simulink model "dig_int_kurt"  (Simulink 6.2)
settings: Solver=ode45  StartTime=0.0  StopTime=1  RelTol=1e-3
undefined symbols (not defined in the file): bit_rev, iBOB, pfb_coeff_gen_calc
libraries: xbsIndex_r3 x1084, casper_library x95, xps_library x32
(part 4 of 8)

== system dig_int_kurt/vacc2/vacc_core2 ==
  note: This BRAM and counter is exactly what is inside the green
      | Delay BRAM block. The functionality was extracted to avoid
      | library issues.
  din : Inport  Port=1  LatchInput=off
  acc_en : Inport  Port=2  LatchInput=off
  Adder : xbsIndex_r3/AddSub  mode=Addition  precision=User Defined  arith_type=Unsigned  n_bits=48  bin_pt=23  quantization=Truncate  overflow=Wrap  latency=2  explicit_period=on  period=1  use_carryin=off  use_carryout=off  en=off  dbl_ovrd=off  show_param=on  use_core=on  pipeline=on  use_rpm=on  gen_core=off
      settings: xl_area=[0, 0, 0, 0, 0, 0, 0]
  BRAM : xbsIndex_r3/Single Port RAM  depth=1024  initVector=0  write_mode=Read Before Write  latency=2  init_zero=on  explicit_period=off  period=1  rst=off  init_reg=0  en=off  dbl_ovrd=off  show_param=off  distributed_mem=off  use_rpm=off  gen_core=off
      settings: xl_area=[0, 0, 0, 0, 0, 0, 0]
  Constant : xbsIndex_r3/Constant  const=0  equ=P=C  arith_type=Unsigned  n_bits=1  bin_pt=0  opselect=C  inp2=PCIN>>17  opr=+  inp1=P  carry=CIN  iostate=0  explicit_period=off  period=1  dbl_ovrd=off
  Constant2 : xbsIndex_r3/Constant  const=1  equ=P=C  arith_type=Boolean  n_bits=1  bin_pt=0  opselect=C  inp2=PCIN>>17  opr=+  inp1=P  carry=CIN  iostate=0  explicit_period=on  period=1  dbl_ovrd=off
  Counter : xbsIndex_r3/Counter  cnt_type=Count Limited  n_bits=10  bin_pt=0  arith_type=Unsigned  start_count=0  cnt_to=1018  cnt_by_val=1  operation=Up  explicit_period=off  period=1  load_pin=off  rst=off  en=off  dbl_ovrd=off  show_param=off  use_rpm=off  gen_core=on
      settings: xl_area=[0, 0, 0, 0, 0, 0, 0]
  Mux : xbsIndex_r3/Mux  inputs=2  precision=Full  arith_type="Signed  (2's comp)"  n_bits=8  bin_pt=2  quantization=Truncate  overflow=Wrap  latency=1  explicit_period=off  period=1  en=off  dbl_ovrd=off  show_param=on  mux_type=off  use_rpm=on  gen_core=off
      settings: xl_area=[0, 0, 0, 0, 0, 0, 0]
  dout : Outport
  wires:
  acc_en/1 -> Mux/1
  Constant/1 -> Mux/2
  BRAM/1 -> Mux/3
  din/1 -> Adder/1
  Mux/1 -> Adder/2
  Adder/1 -> dout/1, BRAM/2
  Counter/1 -> BRAM/1
  Constant2/1 -> BRAM/3

== system dig_int_kurt/fft/fft_biplex0/biplex_core ==
  pol1 : Inport  Port=1  LatchInput=off
  pol2 : Inport  Port=2  LatchInput=off
  sync : Inport  Port=3  LatchInput=off
  shift : Inport  Port=4  LatchInput=off
  fft_stage_1 : Subsystem  mask(fft_stage_n){FFTSize=10, FFTStage=1, BitWidth=18, use_bram=1, CoeffBram=0, MaxCoeffNum=16, quantization=Truncate, overflow=Wrap, add_latency=3, mult_latency=4, bram_latency=3}
      mask prompts: FFTSize "Size of FFT: (2^? pnts)"; FFTStage "Stage of FFT:"; BitWidth "Output Bitwidth:"; use_bram "Implement Delays in BRAM:"; CoeffBram "Store Coefficients in BRAM:"; MaxCoeffNum "Maximum Coefficient Depth: (2^?)"; quantization "Quantization Behavior"; overflow "Overflow Behavior"; add_latency "Add Latency"; mult_latency "Mult Latency"; bram_latency "BRAM Latency"
      mask init:
      | fft_stage_n_init(gcb,...
      |     'FFTSize', FFTSize,...
      |     'FFTStage', FFTStage,...
      |     'BitWidth', BitWidth,...
      |     'use_bram', use_bram,...
      |     'CoeffBram', CoeffBram,...
      |     'MaxCoeffNum', MaxCoeffNum,...
      |     'quantization', quantization,...
      |     'overflow', overflow,...
      |     'add_latency', add_latency,...
      |     'mult_latency', mult_latency,...
      |     'bram_latency', bram_latency);
      settings: AttributesFormatString=FFTSize=10, FFTStage=1, BitWidth=18
      mask StyleString: edit,edit,edit,edit,edit,edit,popup(Truncate|Round  (unbiased: +/- Inf)|Round  (unbiased: Even Values)),popup(Wrap|Saturate|Error),edit,edit,edit
  fft_stage_10 : Subsystem  AncestorBlock=casper_library/FFTs/fft_stage_n  mask(fft_stage_n){FFTSize=10, FFTStage=10, BitWidth=18, use_bram=0, CoeffBram=1, MaxCoeffNum=16, quantization=Truncate, overflow=Wrap, add_latency=3, mult_latency=4, bram_latency=3}
      mask prompts: FFTSize "Size of FFT: (2^? pnts)"; FFTStage "Stage of FFT:"; BitWidth "Output Bitwidth:"; use_bram "Implement Delays in BRAM:"; CoeffBram "Store Coefficients in BRAM:"; MaxCoeffNum "Maximum Coefficient Depth: (2^?)"; quantization "Quantization Behavior"; overflow "Overflow Behavior"; add_latency "Add Latency"; mult_latency "Mult Latency"; bram_latency "BRAM Latency"
      mask init: same as dig_int_kurt/fft/fft_biplex0/biplex_core/fft_stage_1
      settings: AttributesFormatString=FFTSize=10, FFTStage=10, BitWidth=18
      mask StyleString: edit,edit,edit,edit,edit,edit,popup(Truncate|Round  (unbiased: +/- Inf)|Round  (unbiased: Even Values)),popup(Wrap|Saturate|Error),edit,edit,edit
  fft_stage_2 : Subsystem  AncestorBlock=casper_library/FFTs/fft_stage_n  mask(fft_stage_n){FFTSize=10, FFTStage=2, BitWidth=18, use_bram=1, CoeffBram=0, MaxCoeffNum=16, quantization=Truncate, overflow=Wrap, add_latency=3, mult_latency=4, bram_latency=3}
      mask prompts: FFTSize "Size of FFT: (2^? pnts)"; FFTStage "Stage of FFT:"; BitWidth "Output Bitwidth:"; use_bram "Implement Delays in BRAM:"; CoeffBram "Store Coefficients in BRAM:"; MaxCoeffNum "Maximum Coefficient Depth: (2^?)"; quantization "Quantization Behavior"; overflow "Overflow Behavior"; add_latency "Add Latency"; mult_latency "Mult Latency"; bram_latency "BRAM Latency"
      mask init: same as dig_int_kurt/fft/fft_biplex0/biplex_core/fft_stage_1
      settings: AttributesFormatString=FFTSize=10, FFTStage=2, BitWidth=18
      mask StyleString: edit,edit,edit,edit,edit,edit,popup(Truncate|Round  (unbiased: +/- Inf)|Round  (unbiased: Even Values)),popup(Wrap|Saturate|Error),edit,edit,edit
  fft_stage_3 : Subsystem  AncestorBlock=casper_library/FFTs/fft_stage_n  mask(fft_stage_n){FFTSize=10, FFTStage=3, BitWidth=18, use_bram=1, CoeffBram=0, MaxCoeffNum=16, quantization=Truncate, overflow=Wrap, add_latency=3, mult_latency=4, bram_latency=3}
      mask prompts: FFTSize "Size of FFT: (2^? pnts)"; FFTStage "Stage of FFT:"; BitWidth "Output Bitwidth:"; use_bram "Implement Delays in BRAM:"; CoeffBram "Store Coefficients in BRAM:"; MaxCoeffNum "Maximum Coefficient Depth: (2^?)"; quantization "Quantization Behavior"; overflow "Overflow Behavior"; add_latency "Add Latency"; mult_latency "Mult Latency"; bram_latency "BRAM Latency"
      mask init: same as dig_int_kurt/fft/fft_biplex0/biplex_core/fft_stage_1
      settings: AttributesFormatString=FFTSize=10, FFTStage=3, BitWidth=18
      mask StyleString: edit,edit,edit,edit,edit,edit,popup(Truncate|Round  (unbiased: +/- Inf)|Round  (unbiased: Even Values)),popup(Wrap|Saturate|Error),edit,edit,edit
  fft_stage_4 : Subsystem  AncestorBlock=casper_library/FFTs/fft_stage_n  mask(fft_stage_n){FFTSize=10, FFTStage=4, BitWidth=18, use_bram=1, CoeffBram=0, MaxCoeffNum=16, quantization=Truncate, overflow=Wrap, add_latency=3, mult_latency=4, bram_latency=3}
      mask prompts: FFTSize "Size of FFT: (2^? pnts)"; FFTStage "Stage of FFT:"; BitWidth "Output Bitwidth:"; use_bram "Implement Delays in BRAM:"; CoeffBram "Store Coefficients in BRAM:"; MaxCoeffNum "Maximum Coefficient Depth: (2^?)"; quantization "Quantization Behavior"; overflow "Overflow Behavior"; add_latency "Add Latency"; mult_latency "Mult Latency"; bram_latency "BRAM Latency"
      mask init: same as dig_int_kurt/fft/fft_biplex0/biplex_core/fft_stage_1
      settings: AttributesFormatString=FFTSize=10, FFTStage=4, BitWidth=18
      mask StyleString: edit,edit,edit,edit,edit,edit,popup(Truncate|Round  (unbiased: +/- Inf)|Round  (unbiased: Even Values)),popup(Wrap|Saturate|Error),edit,edit,edit
  fft_stage_5 : Subsystem  AncestorBlock=casper_library/FFTs/fft_stage_n  mask(fft_stage_n){FFTSize=10, FFTStage=5, BitWidth=18, use_bram=0, CoeffBram=0, MaxCoeffNum=16, quantization=Truncate, overflow=Wrap, add_latency=3, mult_latency=4, bram_latency=3}
      mask prompts: FFTSize "Size of FFT: (2^? pnts)"; FFTStage "Stage of FFT:"; BitWidth "Output Bitwidth:"; use_bram "Implement Delays in BRAM:"; CoeffBram "Store Coefficients in BRAM:"; MaxCoeffNum "Maximum Coefficient Depth: (2^?)"; quantization "Quantization Behavior"; overflow "Overflow Behavior"; add_latency "Add Latency"; mult_latency "Mult Latency"; bram_latency "BRAM Latency"
      mask init: same as dig_int_kurt/fft/fft_biplex0/biplex_core/fft_stage_1
      settings: AttributesFormatString=FFTSize=10, FFTStage=5, BitWidth=18
      mask StyleString: edit,edit,edit,edit,edit,edit,popup(Truncate|Round  (unbiased: +/- Inf)|Round  (unbiased: Even Values)),popup(Wrap|Saturate|Error),edit,edit,edit
  fft_stage_6 : Subsystem  AncestorBlock=casper_library/FFTs/fft_stage_n  mask(fft_stage_n){FFTSize=10, FFTStage=6, BitWidth=18, use_bram=0, CoeffBram=0, MaxCoeffNum=16, quantization=Truncate, overflow=Wrap, add_latency=3, mult_latency=4, bram_latency=3}
      mask prompts: FFTSize "Size of FFT: (2^? pnts)"; FFTStage "Stage of FFT:"; BitWidth "Output Bitwidth:"; use_bram "Implement Delays in BRAM:"; CoeffBram "Store Coefficients in BRAM:"; MaxCoeffNum "Maximum Coefficient Depth: (2^?)"; quantization "Quantization Behavior"; overflow "Overflow Behavior"; add_latency "Add Latency"; mult_latency "Mult Latency"; bram_latency "BRAM Latency"
      mask init: same as dig_int_kurt/fft/fft_biplex0/biplex_core/fft_stage_1
      settings: AttributesFormatString=FFTSize=10, FFTStage=6, BitWidth=18
      mask StyleString: edit,edit,edit,edit,edit,edit,popup(Truncate|Round  (unbiased: +/- Inf)|Round  (unbiased: Even Values)),popup(Wrap|Saturate|Error),edit,edit,edit
  fft_stage_7 : Subsystem  AncestorBlock=casper_library/FFTs/fft_stage_n  mask(fft_stage_n){FFTSize=10, FFTStage=7, BitWidth=18, use_bram=0, CoeffBram=0, MaxCoeffNum=16, quantization=Truncate, overflow=Wrap, add_latency=3, mult_latency=4, bram_latency=3}
      mask prompts: FFTSize "Size of FFT: (2^? pnts)"; FFTStage "Stage of FFT:"; BitWidth "Output Bitwidth:"; use_bram "Implement Delays in BRAM:"; CoeffBram "Store Coefficients in BRAM:"; MaxCoeffNum "Maximum Coefficient Depth: (2^?)"; quantization "Quantization Behavior"; overflow "Overflow Behavior"; add_latency "Add Latency"; mult_latency "Mult Latency"; bram_latency "BRAM Latency"
      mask init: same as dig_int_kurt/fft/fft_biplex0/biplex_core/fft_stage_1
      settings: AttributesFormatString=FFTSize=10, FFTStage=7, BitWidth=18
      mask StyleString: edit,edit,edit,edit,edit,edit,popup(Truncate|Round  (unbiased: +/- Inf)|Round  (unbiased: Even Values)),popup(Wrap|Saturate|Error),edit,edit,edit
  fft_stage_8 : Subsystem  AncestorBlock=casper_library/FFTs/fft_stage_n  mask(fft_stage_n){FFTSize=10, FFTStage=8, BitWidth=18, use_bram=0, CoeffBram=1, MaxCoeffNum=16, quantization=Truncate, overflow=Wrap, add_latency=3, mult_latency=4, bram_latency=3}
      mask prompts: FFTSize "Size of FFT: (2^? pnts)"; FFTStage "Stage of FFT:"; BitWidth "Output Bitwidth:"; use_bram "Implement Delays in BRAM:"; CoeffBram "Store Coefficients in BRAM:"; MaxCoeffNum "Maximum Coefficient Depth: (2^?)"; quantization "Quantization Behavior"; overflow "Overflow Behavior"; add_latency "Add Latency"; mult_latency "Mult Latency"; bram_latency "BRAM Latency"
      mask init: same as dig_int_kurt/fft/fft_biplex0/biplex_core/fft_stage_1
      settings: AttributesFormatString=FFTSize=10, FFTStage=8, BitWidth=18
      mask StyleString: edit,edit,edit,edit,edit,edit,popup(Truncate|Round  (unbiased: +/- Inf)|Round  (unbiased: Even Values)),popup(Wrap|Saturate|Error),edit,edit,edit
  fft_stage_9 : Subsystem  AncestorBlock=casper_library/FFTs/fft_stage_n  mask(fft_stage_n){FFTSize=10, FFTStage=9, BitWidth=18, use_bram=0, CoeffBram=1, MaxCoeffNum=16, quantization=Truncate, overflow=Wrap, add_latency=3, mult_latency=4, bram_latency=3}
      mask prompts: FFTSize "Size of FFT: (2^? pnts)"; FFTStage "Stage of FFT:"; BitWidth "Output Bitwidth:"; use_bram "Implement Delays in BRAM:"; CoeffBram "Store Coefficients in BRAM:"; MaxCoeffNum "Maximum Coefficient Depth: (2^?)"; quantization "Quantization Behavior"; overflow "Overflow Behavior"; add_latency "Add Latency"; mult_latency "Mult Latency"; bram_latency "BRAM Latency"
      mask init: same as dig_int_kurt/fft/fft_biplex0/biplex_core/fft_stage_1
      settings: AttributesFormatString=FFTSize=10, FFTStage=9, BitWidth=18
      mask StyleString: edit,edit,edit,edit,edit,edit,popup(Truncate|Round  (unbiased: +/- Inf)|Round  (unbiased: Even Values)),popup(Wrap|Saturate|Error),edit,edit,edit
  out1 : Outport
  out2 : Outport  Port=2
  of : Outport  Port=3
  sync_out : Outport  Port=4
  wires:
  fft_stage_1/1(out1) -> fft_stage_2/1(in1)
  fft_stage_1/2(out2) -> fft_stage_2/2(in2)
  fft_stage_1/3(of) -> fft_stage_2/3(of_in)
  fft_stage_1/4(sync_out) -> fft_stage_2/4(sync)
  shift/1 -> fft_stage_2/5(shift), fft_stage_3/5(shift), fft_stage_4/5(shift), fft_stage_5/5(shift), fft_stage_6/5(shift), fft_stage_7/5(shift), fft_stage_8/5(shift), fft_stage_9/5(shift), fft_stage_10/5(shift), fft_stage_1/4(shift)
  fft_stage_2/1(out1) -> fft_stage_3/1(in1)
  fft_stage_2/2(out2) -> fft_stage_3/2(in2)
  fft_stage_2/3(of) -> fft_stage_3/3(of_in)
  fft_stage_2/4(sync_out) -> fft_stage_3/4(sync)
  fft_stage_3/1(out1) -> fft_stage_4/1(in1)
  fft_stage_3/2(out2) -> fft_stage_4/2(in2)
  fft_stage_3/3(of) -> fft_stage_4/3(of_in)
  fft_stage_3/4(sync_out) -> fft_stage_4/4(sync)
  fft_stage_4/1(out1) -> fft_stage_5/1(in1)
  fft_stage_4/2(out2) -> fft_stage_5/2(in2)
  fft_stage_4/3(of) -> fft_stage_5/3(of_in)
  fft_stage_4/4(sync_out) -> fft_stage_5/4(sync)
  fft_stage_5/1(out1) -> fft_stage_6/1(in1)
  fft_stage_5/2(out2) -> fft_stage_6/2(in2)
  fft_stage_5/3(of) -> fft_stage_6/3(of_in)
  fft_stage_5/4(sync_out) -> fft_stage_6/4(sync)
  fft_stage_6/1(out1) -> fft_stage_7/1(in1)
  fft_stage_6/2(out2) -> fft_stage_7/2(in2)
  fft_stage_6/3(of) -> fft_stage_7/3(of_in)
  fft_stage_6/4(sync_out) -> fft_stage_7/4(sync)
  fft_stage_7/1(out1) -> fft_stage_8/1(in1)
  fft_stage_7/2(out2) -> fft_stage_8/2(in2)
  fft_stage_7/3(of) -> fft_stage_8/3(of_in)
  fft_stage_7/4(sync_out) -> fft_stage_8/4(sync)
  fft_stage_8/1(out1) -> fft_stage_9/1(in1)
  fft_stage_8/2(out2) -> fft_stage_9/2(in2)
  fft_stage_8/3(of) -> fft_stage_9/3(of_in)
  fft_stage_8/4(sync_out) -> fft_stage_9/4(sync)
  fft_stage_9/1(out1) -> fft_stage_10/1(in1)
  fft_stage_9/2(out2) -> fft_stage_10/2(in2)
  fft_stage_9/3(of) -> fft_stage_10/3(of_in)
  fft_stage_9/4(sync_out) -> fft_stage_10/4(sync)
  pol1/1 -> fft_stage_1/1(in1)
  pol2/1 -> fft_stage_1/2(in2)
  sync/1 -> fft_stage_1/3(sync)
  fft_stage_10/1(out1) -> out1/1
  fft_stage_10/2(out2) -> out2/1
  fft_stage_10/3(of) -> of/1
  fft_stage_10/4(sync_out) -> sync_out/1

== system dig_int_kurt/fft/fft_biplex0/biplex_cplx_unscrambler ==
  even : Inport  Port=1  LatchInput=off
  odd : Inport  Port=2  LatchInput=off
  sync : Inport  Port=3  LatchInput=off
  Constant : xbsIndex_r3/Constant  const=1  equ=P=C  arith_type=Boolean  n_bits=1  bin_pt=0  opselect=C  inp2=PCIN>>17  opr=+  inp1=P  carry=CIN  iostate=0  explicit_period=on  period=1  dbl_ovrd=off
  Constant1 : xbsIndex_r3/Constant  const=2^(FFTSize-1)  equ=P=C  arith_type=Unsigned  n_bits=FFTSize  bin_pt=0  opselect=C  inp2=PCIN>>17  opr=+  inp1=P  carry=CIN  iostate=0  explicit_period=on  period=1  dbl_ovrd=off
  Constant2 : xbsIndex_r3/Constant  const=2^(FFTSize-1)  equ=P=C  arith_type=Unsigned  n_bits=FFTSize  bin_pt=0  opselect=C  inp2=PCIN>>17  opr=+  inp1=P  carry=CIN  iostate=0  explicit_period=on  period=1  dbl_ovrd=off
  Convert : xbsIndex_r3/Convert  arith_type=Unsigned  n_bits=1  bin_pt=0  quantization=Truncate  overflow=Wrap  latency=0  explicit_period=off  period=1  dbl_ovrd=off  show_param=off  inserted_by_tool=off  pipeline=off
      settings: xl_area=[0, 0, 0, 0, 0, 0, 0]
  Convert1 : xbsIndex_r3/Convert  arith_type=Unsigned  n_bits=1  bin_pt=0  quantization=Truncate  overflow=Wrap  latency=0  explicit_period=off  period=1  dbl_ovrd=off  show_param=off  inserted_by_tool=off  pipeline=off
      settings: xl_area=[0, 0, 0, 0, 0, 0, 0]
  Counter : xbsIndex_r3/Counter  cnt_type=Free Running  n_bits=FFTSize  bin_pt=0  arith_type=Unsigned  start_count=0  cnt_to=Inf  cnt_by_val=1  operation=Up  explicit_period=off  period=1  load_pin=off  rst=on  en=off  dbl_ovrd=off  show_param=off  use_rpm=on  gen_core=off
      settings: xl_area=[0, 0, 0, 0, 0, 0, 0]
  Counter1 : xbsIndex_r3/Counter  cnt_type=Free Running  n_bits=FFTSize  bin_pt=0  arith_type=Unsigned  start_count=0  cnt_to=Inf  cnt_by_val=1  operation=Up  explicit_period=off  period=1  load_pin=off  rst=on  en=off  dbl_ovrd=off  show_param=off  use_rpm=on  gen_core=off
      settings: xl_area=[0, 0, 0, 0, 0, 0, 0]
  Relational : xbsIndex_r3/Relational  mode=a<=b  latency=0  explicit_period=off  period=1  en=off  dbl_ovrd=off  show_param=off
      settings: xl_area=[0, 0, 0, 0, 0, 0, 0]
  Relational1 : xbsIndex_r3/Relational  mode=a<=b  latency=0  explicit_period=off  period=1  en=off  dbl_ovrd=off  show_param=off
      settings: xl_area=[0, 0, 0, 0, 0, 0, 0]
  barrel_switcher : Subsystem  AncestorBlock=casper_library/Reorder/barrel_switcher  mask(barrel_switcher){n_inputs=1}
      mask prompts: n_inputs "Number of Inputs: (2^?)"
      mask init:
      | barrel_switcher_init(gcb,...
      |     'n_inputs', n_inputs);
      settings: AttributesFormatString=n_inputs=1
  barrel_switcher1 : Subsystem  AncestorBlock=casper_library/Reorder/barrel_switcher  mask(barrel_switcher){n_inputs=1}
      mask prompts: n_inputs "Number of Inputs: (2^?)"
      mask init:
      | barrel_switcher_init(gcb,...
      |     'n_inputs', n_inputs);
      settings: AttributesFormatString=n_inputs=1
  reorder : Subsystem  AncestorBlock=casper_library/Reorder/reorder  mask(reorder){map=[0 256 128 384 64 320 192 448 32 288 160 416 96 352 224 480 16 272 144 400 80 336 208 464 48 304 176 432 112 368 240 496 8 264 136 392 72 328 200 456 40 296 168 424 104 360 232 488 24 280 152 408 88 344 216 472 56 312 184 440 120 376 248 504 4 260 132 388 68 324 196 452 36 292 164 420 100 356 228 484 20 276 148 404 84 340 212 468 52 308 180 436 116 372 244 500 12 268 140 396 76 332 204 460 44 300 172 428 108 364 236 492 28 284 156 412 92 348 220 476 60 316 188 444 124 380 252 508 2 258 130 386 66 322 194 450 34 290 162 418 98 354 226 482 18 274 146 402 82 338 210 466 50 306 178 434 114 370 242 498 10 266 138 394 74 330 202 458 42 298 170 426 106 362 234 490 26 282 154 410 90 346 218 474 58 314 186 442 122 378 250 506 6 262 134 390 70 326 198 454 38 294 166 422 102 358 230 486 22 278 150 406 86 342 214 470 54 310 182 438 118 374 246 502 14 270 142 398 78 334 206 462 46 302 174 430 110 366 238 494 30 286 158 414 94 350 222 478 62 318 190 446 126 382 254 510 1 257 129 385 65 321 193 449 33 289 161 417 97 353 225 481 17 273 145 401 81 337 209 465 49 305 177 433 113 369 241 497 9 265 137 393 73 329 201 457 41 297 169 425 105 361 233 489 25 281 153 409 89 345 217 473 57 313 185 441 121 377 249 505 5 261 133 389 69 325 197 453 37 293 165 421 101 357 229 485 21 277 149 405 85 341 213 469 53 309 181 437 117 373 245 501 13 269 141 397 77 333 205 461 45 301 173 429 109 365 237 493 29 285 157 413 93 349 221 477 61 317 189 445 125 381 253 509 3 259 131 387 67 323 195 451 35 291 163 419 99 355 227 483 19 275 147 403 83 339 211 467 51 307 179 435 115 371 243 499 11 267 139 395 75 331 203 459 43 299 171 427 107 363 235 491 27 283 155 411 91 347 219 475 59 315 187 443 123 379 251 507 7 263 135 391 71 327 199 455 39 295 167 423 103 359 231 487 23 279 151 407 87 343 215 471 55 311 183 439 119 375 247 503 15 271 143 399 79 335 207 463 47 303 175 431 111 367 239 495 31 287 159 415 95 351 223 479 63 319 191 447 127 383 255 511 512 768 640 896 576 832 704 960 544 800 672 928 608 864 736 992 528 784 656 912 592 848 720 976 560 816 688 944 624 880 752 1008 520 776 648 904 584 840 712 968 552 808 680 936 616 872 744 1000 536 792 664 920 600 856 728 984 568 824 696 952 632 888 760 1016 516 772 644 900 580 836 708 964 548 804 676 932 612 868 740 996 532 788 660 916 596 852 724 980 564 820 692 948 628 884 756 1012 524 780 652 908 588 844 716 972 556 812 684 940 620 876 748 1004 540 796 668 924 604 860 732 988 572 828 700 956 636 892 764 1020 514 770 642 898 578 834 706 962 546 802 674 930 610 866 738 994 530 786 658 914 594 850 722 978 562 818 690 946 626 882 754 1010 522 778 650 906 586 842 714 970 554 810 682 938 618 874 746 1002 538 794 666 922 602 858 730 986 570 826 698 954 634 890 762 1018 518 774 646 902 582 838 710 966 550 806 678 934 614 870 742 998 534 790 662 918 598 854 726 982 566 822 694 950 630 886 758 1014 526 782 654 910 590 846 718 974 558 814 686 942 622 878 750 1006 542 798 670 926 606 862 734 990 574 830 702 958 638 894 766 1022 513 769 641 897 577 833 705 961 545 801 673 929 609 865 737 993 529 785 657 913 593 849 721 977 561 817 689 945 625 881 753 1009 521 777 649 905 585 841 713 969 553 809 681 937 617 873 745 1001 537 793 665 921 601 857 729 985 569 825 697 953 633 889 761 1017 517 773 645 901 581 837 709 965 549 805 677 933 613 869 741 997 533 789 661 917 597 853 725 981 565 821 693 949 629 885 757 1013 525 781 653 909 589 845 717 973 557 813 685 941 621 877 749 1005 541 797 669 925 605 861 733 989 573 829 701 957 637 893 765 1021 515 771 643 899 579 835 707 963 547 803 675 931 611 867 739 995 531 787 659 915 595 851 723 979 563 819 691 947 627 883 755 1011 523 779 651 907 587 843 715 971 555 811 683 939 619 875 747 1003 539 795 667 923 603 859 731 987 571 827 699 955 635 891 763 1019 519 775 647 903 583 839 711 967 551 807 679 935 615 871 743 999 535 791 663 919 599 855 727 983 567 823 695 951 631 887 759 1015 527 783 655 911 591 847 719 975 559 815 687 943 623 879 751 1007 543 799 671 927 607 863 735 991 575 831 703 959 639 895 767 1023], n_inputs=1, bram_latency=3, map_latency=0, double_buffer=0}
      mask prompts: map "Output Order:"; n_inputs "Number of inputs"; bram_latency "BRAM Latency"; map_latency "Map Latency"; double_buffer "Double Buffer"
      mask init:
      | reorder_init(gcb, ...
      |     'map', map, ...
      |     'n_inputs', n_inputs, ...
      |     'bram_latency', bram_latency, ...
      |     'map_latency', map_latency, ...
      |     'double_buffer', double_buffer);
      settings: AttributesFormatString=order=2
  reorder1 : Subsystem  AncestorBlock=casper_library/Reorder/reorder  mask(reorder){map=[512 768 640 896 576 832 704 960 544 800 672 928 608 864 736 992 528 784 656 912 592 848 720 976 560 816 688 944 624 880 752 1008 520 776 648 904 584 840 712 968 552 808 680 936 616 872 744 1000 536 792 664 920 600 856 728 984 568 824 696 952 632 888 760 1016 516 772 644 900 580 836 708 964 548 804 676 932 612 868 740 996 532 788 660 916 596 852 724 980 564 820 692 948 628 884 756 1012 524 780 652 908 588 844 716 972 556 812 684 940 620 876 748 1004 540 796 668 924 604 860 732 988 572 828 700 956 636 892 764 1020 514 770 642 898 578 834 706 962 546 802 674 930 610 866 738 994 530 786 658 914 594 850 722 978 562 818 690 946 626 882 754 1010 522 778 650 906 586 842 714 970 554 810 682 938 618 874 746 1002 538 794 666 922 602 858 730 986 570 826 698 954 634 890 762 1018 518 774 646 902 582 838 710 966 550 806 678 934 614 870 742 998 534 790 662 918 598 854 726 982 566 822 694 950 630 886 758 1014 526 782 654 910 590 846 718 974 558 814 686 942 622 878 750 1006 542 798 670 926 606 862 734 990 574 830 702 958 638 894 766 1022 513 769 641 897 577 833 705 961 545 801 673 929 609 865 737 993 529 785 657 913 593 849 721 977 561 817 689 945 625 881 753 1009 521 777 649 905 585 841 713 969 553 809 681 937 617 873 745 1001 537 793 665 921 601 857 729 985 569 825 697 953 633 889 761 1017 517 773 645 901 581 837 709 965 549 805 677 933 613 869 741 997 533 789 661 917 597 853 725 981 565 821 693 949 629 885 757 1013 525 781 653 909 589 845 717 973 557 813 685 941 621 877 749 1005 541 797 669 925 605 861 733 989 573 829 701 957 637 893 765 1021 515 771 643 899 579 835 707 963 547 803 675 931 611 867 739 995 531 787 659 915 595 851 723 979 563 819 691 947 627 883 755 1011 523 779 651 907 587 843 715 971 555 811 683 939 619 875 747 1003 539 795 667 923 603 859 731 987 571 827 699 955 635 891 763 1019 519 775 647 903 583 839 711 967 551 807 679 935 615 871 743 999 535 791 663 919 599 855 727 983 567 823 695 951 631 887 759 1015 527 783 655 911 591 847 719 975 559 815 687 943 623 879 751 1007 543 799 671 927 607 863 735 991 575 831 703 959 639 895 767 1023 0 256 128 384 64 320 192 448 32 288 160 416 96 352 224 480 16 272 144 400 80 336 208 464 48 304 176 432 112 368 240 496 8 264 136 392 72 328 200 456 40 296 168 424 104 360 232 488 24 280 152 408 88 344 216 472 56 312 184 440 120 376 248 504 4 260 132 388 68 324 196 452 36 292 164 420 100 356 228 484 20 276 148 404 84 340 212 468 52 308 180 436 116 372 244 500 12 268 140 396 76 332 204 460 44 300 172 428 108 364 236 492 28 284 156 412 92 348 220 476 60 316 188 444 124 380 252 508 2 258 130 386 66 322 194 450 34 290 162 418 98 354 226 482 18 274 146 402 82 338 210 466 50 306 178 434 114 370 242 498 10 266 138 394 74 330 202 458 42 298 170 426 106 362 234 490 26 282 154 410 90 346 218 474 58 314 186 442 122 378 250 506 6 262 134 390 70 326 198 454 38 294 166 422 102 358 230 486 22 278 150 406 86 342 214 470 54 310 182 438 118 374 246 502 14 270 142 398 78 334 206 462 46 302 174 430 110 366 238 494 30 286 158 414 94 350 222 478 62 318 190 446 126 382 254 510 1 257 129 385 65 321 193 449 33 289 161 417 97 353 225 481 17 273 145 401 81 337 209 465 49 305 177 433 113 369 241 497 9 265 137 393 73 329 201 457 41 297 169 425 105 361 233 489 25 281 153 409 89 345 217 473 57 313 185 441 121 377 249 505 5 261 133 389 69 325 197 453 37 293 165 421 101 357 229 485 21 277 149 405 85 341 213 469 53 309 181 437 117 373 245 501 13 269 141 397 77 333 205 461 45 301 173 429 109 365 237 493 29 285 157 413 93 349 221 477 61 317 189 445 125 381 253 509 3 259 131 387 67 323 195 451 35 291 163 419 99 355 227 483 19 275 147 403 83 339 211 467 51 307 179 435 115 371 243 499 11 267 139 395 75 331 203 459 43 299 171 427 107 363 235 491 27 283 155 411 91 347 219 475 59 315 187 443 123 379 251 507 7 263 135 391 71 327 199 455 39 295 167 423 103 359 231 487 23 279 151 407 87 343 215 471 55 311 183 439 119 375 247 503 15 271 143 399 79 335 207 463 47 303 175 431 111 367 239 495 31 287 159 415 95 351 223 479 63 319 191 447 127 383 255 511], n_inputs=1, bram_latency=3, map_latency=0, double_buffer=0}
      mask prompts: map "Output Order:"; n_inputs "Number of inputs"; bram_latency "BRAM Latency"; map_latency "Map Latency"; double_buffer "Double Buffer"
      mask init:
      | reorder_init(gcb, ...
      |     'map', map, ...
      |     'n_inputs', n_inputs, ...
      |     'bram_latency', bram_latency, ...
      |     'map_latency', map_latency, ...
      |     'double_buffer', double_buffer);
      settings: AttributesFormatString=order=2
  pol1 : Outport
  pol2 : Outport  Port=2
  sync_out : Outport  Port=3
  wires:
  Convert/1 -> barrel_switcher/1(sel)
  Convert1/1 -> barrel_switcher1/1(sel)
  Relational1/1 -> Convert1/1
  Relational/1 -> Convert/1
  Constant2/1 -> Relational1/1
  Counter1/1 -> Relational1/2
  Counter/1 -> Relational/2
  Constant1/1 -> Relational/1
  Constant/1 -> reorder1/2(en), reorder/2(en)
  sync/1 -> Counter/1, barrel_switcher/2(sync_in)
  barrel_switcher1/3(Out2) -> pol2/1
  barrel_switcher1/2(Out1) -> pol1/1
  barrel_switcher1/1(sync_out) -> sync_out/1
  odd/1 -> barrel_switcher/4(In2)
  even/1 -> barrel_switcher/3(In1)
  reorder1/3(dout0) -> barrel_switcher1/4(In2)
  reorder/3(dout0) -> barrel_switcher1/3(In1)
  reorder/1(sync_out) -> Counter1/1, barrel_switcher1/2(sync_in)
  barrel_switcher/3(Out2) -> reorder1/3(din0)
  barrel_switcher/2(Out1) -> reorder/3(din0)
  barrel_switcher/1(sync_out) -> reorder1/1(sync), reorder/1(sync)

== system dig_int_kurt/pfb_fir/pol1_in1_first_tap/delay ==
  In1 : Inport  Port=1  LatchInput=off
  delay_bram : casper_library/Delays/delay_bram  DelayLen=2^(PFBSize-n_inputs)  bram_latency=bram_latency
  Out1 : Outport
  wires:
  In1/1 -> delay_bram/1
  delay_bram/1 -> Out1/1

== system dig_int_kurt/pfb_fir/pol1_in1_first_tap/pfb_coeff_gen ==
  din : Inport  Port=1  LatchInput=off
  sync : Inport  Port=2  LatchInput=off
  Concat : xbsIndex_r3/Concat  num_inputs=4  explicit_period=off  period=1  dbl_ovrd=off
  Counter : xbsIndex_r3/Counter  cnt_type=Free Running  n_bits=10  bin_pt=0  arith_type=Unsigned  start_count=0  cnt_to=Inf  cnt_by_val=1  operation=Up  explicit_period=on  period=1  load_pin=off  rst=on  en=off  dbl_ovrd=off  show_param=off  use_rpm=on  gen_core=off
      settings: xl_area=[0, 0, 0, 0, 0, 0, 0]
  Delay : xbsIndex_r3/Delay  latency=bram_latency+1  reg_retiming=off  explicit_period=off  period=1  en=off  accept_only_valid=off  init_zero=on  dbl_ovrd=off  show_param=off
      settings: xl_area=[0, 0, 0, 0, 0, 0, 0]
  Delay1 : xbsIndex_r3/Delay  latency=4  reg_retiming=off  explicit_period=off  period=1  en=off  accept_only_valid=off  init_zero=on  dbl_ovrd=off  show_param=off
      settings: xl_area=[0, 0, 0, 0, 0, 0, 0]
  ROM1 : xbsIndex_r3/ROM  depth=1024  initVector=pfb_coeff_gen_calc(10, 4,'hamming',0, 0,1,1)  arith_type="Signed  (2's comp)"  n_bits=8  bin_pt=7  latency=3  init_zero=on  explicit_period=off  period=1  rst=off  init_reg=0  en=off  dbl_ovrd=off  show_param=on  distributed_mem=on  use_rpm=on  gen_core=off
      settings: xl_area=[0, 0, 0, 0, 0, 0, 0]
  ROM2 : xbsIndex_r3/ROM  depth=1024  initVector=pfb_coeff_gen_calc(10, 4,'hamming',0, 0,1,2)  arith_type="Signed  (2's comp)"  n_bits=8  bin_pt=7  latency=3  init_zero=on  explicit_period=off  period=1  rst=off  init_reg=0  en=off  dbl_ovrd=off  show_param=on  distributed_mem=on  use_rpm=on  gen_core=off
      settings: xl_area=[0, 0, 0, 0, 0, 0, 0]
  ROM3 : xbsIndex_r3/ROM  depth=1024  initVector=pfb_coeff_gen_calc(10, 4,'hamming',0, 0,1,3)  arith_type="Signed  (2's comp)"  n_bits=8  bin_pt=7  latency=3  init_zero=on  explicit_period=off  period=1  rst=off  init_reg=0  en=off  dbl_ovrd=off  show_param=off  distributed_mem=on  use_rpm=on  gen_core=off
      settings: xl_area=[0, 0, 0, 0, 0, 0, 0]
  ROM4 : xbsIndex_r3/ROM  depth=1024  initVector=pfb_coeff_gen_calc(10, 4,'hamming',0, 0,1,4)  arith_type="Signed  (2's comp)"  n_bits=8  bin_pt=7  latency=3  init_zero=on  explicit_period=off  period=1  rst=off  init_reg=0  en=off  dbl_ovrd=off  show_param=off  distributed_mem=on  use_rpm=on  gen_core=off
      settings: xl_area=[0, 0, 0, 0, 0, 0, 0]
  Register : xbsIndex_r3/Register  init=0  reg_only_valid=off  explicit_period=off  period=1  rst=off  en=off  out_en=off  dbl_ovrd=off  show_param=off
      settings: xl_area=[0, 0, 0, 0, 0, 0, 0]
  Reinterpret{1..4} (4 alike) : xbsIndex_r3/Reinterpret  force_arith_type=on  arith_type=Unsigned  force_bin_pt=on  bin_pt=0  force_valid=on
  dout : Outport
  sync_out : Outport  Port=2
  coeff : Outport  Port=3
  wires:
  din/1 -> Delay1/1
  Delay1/1 -> dout/1
  sync/1 -> Counter/1, Delay/1
  Delay/1 -> sync_out/1
  Concat/1 -> Register/1
  Register/1 -> coeff/1
  Counter/1 -> ROM1/1, ROM2/1, ROM3/1, ROM4/1
  ROM1/1 -> Reinterpret1/1
  Reinterpret1/1 -> Concat/1
  ROM2/1 -> Reinterpret2/1
  Reinterpret2/1 -> Concat/2
  ROM3/1 -> Reinterpret3/1
  Reinterpret3/1 -> Concat/3
  ROM4/1 -> Reinterpret4/1
  Reinterpret4/1 -> Concat/4

== system dig_int_kurt/pfb_fir/pol1_in1_first_tap/ri_to_c ==
  re : Inport  Port=1  LatchInput=off
  im : Inport  Port=2  LatchInput=off
  Concat : xbsIndex_r3/Concat  num_inputs=2  explicit_period=off  period=1  dbl_ovrd=off
  Reinterpret : xbsIndex_r3/Reinterpret  force_arith_type=on  arith_type=Unsigned  force_bin_pt=on  bin_pt=0  force_valid=on
  Reinterpret1 : xbsIndex_r3/Reinterpret  force_arith_type=on  arith_type=Unsigned  force_bin_pt=on  bin_pt=0  force_valid=on
  c : Outport
  wires:
  Reinterpret/1 -> Concat/1
  Reinterpret1/1 -> Concat/2
  re/1 -> Reinterpret/1
  Concat/1 -> c/1
  im/1 -> Reinterpret1/1

== system dig_int_kurt/pfb_fir/pol1_in1_last_tap/pfb_add_tree ==
  din : Inport  Port=1  LatchInput=off
  sync : Inport  Port=2  LatchInput=off
  Reint0_1 : xbsIndex_r3/Reinterpret  force_arith_type=on  arith_type="Signed  (2's comp)"  force_bin_pt=on  bin_pt=14  force_valid=on
  Reint0_2 : xbsIndex_r3/Reinterpret  force_arith_type=on  arith_type="Signed  (2's comp)"  force_bin_pt=on  bin_pt=14  force_valid=on
  Reint1_1 : xbsIndex_r3/Reinterpret  force_arith_type=on  arith_type="Signed  (2's comp)"  force_bin_pt=on  bin_pt=14  force_valid=on
  Reint1_2 : xbsIndex_r3/Reinterpret  force_arith_type=on  arith_type="Signed  (2's comp)"  force_bin_pt=on  bin_pt=14  force_valid=on
  Reint2_1 : xbsIndex_r3/Reinterpret  force_arith_type=on  arith_type="Signed  (2's comp)"  force_bin_pt=on  bin_pt=14  force_valid=on
  Reint2_2 : xbsIndex_r3/Reinterpret  force_arith_type=on  arith_type="Signed  (2's comp)"  force_bin_pt=on  bin_pt=14  force_valid=on
  Reint3_1 : xbsIndex_r3/Reinterpret  force_arith_type=on  arith_type="Signed  (2's comp)"  force_bin_pt=on  bin_pt=14  force_valid=on
  Reint3_2 : xbsIndex_r3/Reinterpret  force_arith_type=on  arith_type="Signed  (2's comp)"  force_bin_pt=on  bin_pt=14  force_valid=on
  Slice0_1 : xbsIndex_r3/Slice  mode=Upper Bit Location + Width  nbits=16  bit1=0  base1=MSB of Input  bit0=0  base0=MSB of Input  boolean_output=off  explicit_period=off  period=1  dbl_ovrd=off
  Slice0_2 : xbsIndex_r3/Slice  mode=Upper Bit Location + Width  nbits=16  bit1=-16  base1=MSB of Input  bit0=0  base0=MSB of Input  boolean_output=off  explicit_period=off  period=1  dbl_ovrd=off
  Slice1_1 : xbsIndex_r3/Slice  mode=Upper Bit Location + Width  nbits=16  bit1=-32  base1=MSB of Input  bit0=0  base0=MSB of Input  boolean_output=off  explicit_period=off  period=1  dbl_ovrd=off
  Slice1_2 : xbsIndex_r3/Slice  mode=Upper Bit Location + Width  nbits=16  bit1=-48  base1=MSB of Input  bit0=0  base0=MSB of Input  boolean_output=off  explicit_period=off  period=1  dbl_ovrd=off
  Slice2_1 : xbsIndex_r3/Slice  mode=Upper Bit Location + Width  nbits=16  bit1=-64  base1=MSB of Input  bit0=0  base0=MSB of Input  boolean_output=off  explicit_period=off  period=1  dbl_ovrd=off
  Slice2_2 : xbsIndex_r3/Slice  mode=Upper Bit Location + Width  nbits=16  bit1=-80  base1=MSB of Input  bit0=0  base0=MSB of Input  boolean_output=off  explicit_period=off  period=1  dbl_ovrd=off
  Slice3_1 : xbsIndex_r3/Slice  mode=Upper Bit Location + Width  nbits=16  bit1=-96  base1=MSB of Input  bit0=0  base0=MSB of Input  boolean_output=off  explicit_period=off  period=1  dbl_ovrd=off
  Slice3_2 : xbsIndex_r3/Slice  mode=Upper Bit Location + Width  nbits=16  bit1=-112  base1=MSB of Input  bit0=0  base0=MSB of Input  boolean_output=off  explicit_period=off  period=1  dbl_ovrd=off
  adder_tree1 : Subsystem  AncestorBlock=casper_library/Misc/adder_tree  mask(adder_tree){n_inputs=4, latency=2}
      mask prompts: n_inputs "Number of Inputs"; latency "Add Latency"
      mask help: Sums all inputs using a tree of adds and delays.
      mask init:
      | adder_tree_init(gcb, ...
      |     'n_inputs', n_inputs, ...
      |     'latency', latency);
      settings: AttributesFormatString=latency 4
      mask Help: eval('xlWeb([getenv(''MLIB_ROOT''), ''\doc\html\sp_adder_tree\sp_adder_tree.html''])')
  adder_tree2 : Subsystem  AncestorBlock=casper_library/Misc/adder_tree  mask(adder_tree){n_inputs=4, latency=2}
      mask prompts: n_inputs "Number of Inputs"; latency "Add Latency"
      mask help: Sums all inputs using a tree of adds and delays.
      mask init:
      | adder_tree_init(gcb, ...
      |     'n_inputs', n_inputs, ...
      |     'latency', latency);
      settings: AttributesFormatString=latency 4
      mask Help: eval('xlWeb([getenv(''MLIB_ROOT''), ''\doc\html\sp_adder_tree\sp_adder_tree.html''])')
  convert1 : xbsIndex_r3/Convert  arith_type="Signed  (2's comp)"  n_bits=18  bin_pt=17  quantization=Truncate  overflow=Saturate  latency=2  explicit_period=off  period=1  dbl_ovrd=off  show_param=off  inserted_by_tool=off  pipeline=off
      settings: xl_area=[0, 0, 0, 0, 0, 0, 0]
  convert2 : xbsIndex_r3/Convert  arith_type="Signed  (2's comp)"  n_bits=18  bin_pt=17  quantization=Truncate  overflow=Saturate  latency=2  explicit_period=off  period=1  dbl_ovrd=off  show_param=off  inserted_by_tool=off  pipeline=off
      settings: xl_area=[0, 0, 0, 0, 0, 0, 0]
  delay1 : xbsIndex_r3/Delay  latency=2  reg_retiming=off  explicit_period=off  period=1  en=off  accept_only_valid=off  init_zero=on  dbl_ovrd=off  show_param=off
      settings: xl_area=[0, 0, 0, 0, 0, 0, 0]
  ri_to_c : casper_library/Misc/ri_to_c
  scale1 : xbsIndex_r3/Scale  scale_factor=-3  explicit_period=off  period=1  dbl_ovrd=off
  scale2 : xbsIndex_r3/Scale  scale_factor=-3  explicit_period=off  period=1  dbl_ovrd=off
  dout : Outport
  sync_out : Outport  Port=2
  wires:
  adder_tree1/2(dout) -> scale1/1
  scale1/1 -> convert1/1
  adder_tree2/2(dout) -> scale2/1
  scale2/1 -> convert2/1
  convert1/1 -> ri_to_c/1
  convert2/1 -> ri_to_c/2
  ri_to_c/1 -> dout/1
  sync/1 -> adder_tree1/1(sync), adder_tree2/1(sync)
  adder_tree1/1(sync_out) -> delay1/1
  delay1/1 -> sync_out/1
  din/1 -> Slice0_1/1, Slice0_2/1, Slice1_1/1, Slice1_2/1, Slice2_1/1, Slice2_2/1, Slice3_1/1, Slice3_2/1
  Slice0_1/1 -> Reint0_1/1
  Reint0_1/1 -> adder_tree1/2(din1)
  Slice0_2/1 -> Reint0_2/1
  Reint0_2/1 -> adder_tree2/2(din1)
  Slice1_1/1 -> Reint1_1/1
  Reint1_1/1 -> adder_tree1/3(din2)
  Slice1_2/1 -> Reint1_2/1
  Reint1_2/1 -> adder_tree2/3(din2)
  Slice2_1/1 -> Reint2_1/1
  Reint2_1/1 -> adder_tree1/4(din3)
  Slice2_2/1 -> Reint2_2/1
  Reint2_2/1 -> adder_tree2/4(din3)
  Slice3_1/1 -> Reint3_1/1
  Reint3_1/1 -> adder_tree1/5(din4)
  Slice3_2/1 -> Reint3_2/1
  Reint3_2/1 -> adder_tree2/5(din4)

== system dig_int_kurt/pfb_fir/pol1_in1_last_tap/ri_to_c ==
  re : Inport  Port=1  LatchInput=off
  im : Inport  Port=2  LatchInput=off
  Concat : xbsIndex_r3/Concat  num_inputs=2  explicit_period=off  period=1  dbl_ovrd=off
  Reinterpret : xbsIndex_r3/Reinterpret  force_arith_type=on  arith_type=Unsigned  force_bin_pt=on  bin_pt=0  force_valid=on
  Reinterpret1 : xbsIndex_r3/Reinterpret  force_arith_type=on  arith_type=Unsigned  force_bin_pt=on  bin_pt=0  force_valid=on
  c : Outport
  wires:
  im/1 -> Reinterpret1/1
  Concat/1 -> c/1
  re/1 -> Reinterpret/1
  Reinterpret1/1 -> Concat/2
  Reinterpret/1 -> Concat/1

== system dig_int_kurt/pfb_fir/pol2_in1_first_tap/delay ==
  In1 : Inport  Port=1  LatchInput=off
  delay_bram : casper_library/Delays/delay_bram  DelayLen=2^(PFBSize-n_inputs)  bram_latency=bram_latency
  Out1 : Outport
  wires:
  In1/1 -> delay_bram/1
  delay_bram/1 -> Out1/1

== system dig_int_kurt/pfb_fir/pol2_in1_first_tap/pfb_coeff_gen ==
  din : Inport  Port=1  LatchInput=off
  sync : Inport  Port=2  LatchInput=off
  Concat : xbsIndex_r3/Concat  num_inputs=4  explicit_period=off  period=1  dbl_ovrd=off
  Counter : xbsIndex_r3/Counter  cnt_type=Free Running  n_bits=10  bin_pt=0  arith_type=Unsigned  start_count=0  cnt_to=Inf  cnt_by_val=1  operation=Up  explicit_period=on  period=1  load_pin=off  rst=on  en=off  dbl_ovrd=off  show_param=off  use_rpm=on  gen_core=off
      settings: xl_area=[0, 0, 0, 0, 0, 0, 0]
  Delay : xbsIndex_r3/Delay  latency=bram_latency+1  reg_retiming=off  explicit_period=off  period=1  en=off  accept_only_valid=off  init_zero=on  dbl_ovrd=off  show_param=off
      settings: xl_area=[0, 0, 0, 0, 0, 0, 0]
  Delay1 : xbsIndex_r3/Delay  latency=4  reg_retiming=off  explicit_period=off  period=1  en=off  accept_only_valid=off  init_zero=on  dbl_ovrd=off  show_param=off
      settings: xl_area=[0, 0, 0, 0, 0, 0, 0]
  ROM1 : xbsIndex_r3/ROM  depth=1024  initVector=pfb_coeff_gen_calc(10, 4,'hamming',0, 0,1,1)  arith_type="Signed  (2's comp)"  n_bits=8  bin_pt=7  latency=3  init_zero=on  explicit_period=off  period=1  rst=off  init_reg=0  en=off  dbl_ovrd=off  show_param=on  distributed_mem=on  use_rpm=on  gen_core=off
      settings: xl_area=[0, 0, 0, 0, 0, 0, 0]
  ROM2 : xbsIndex_r3/ROM  depth=1024  initVector=pfb_coeff_gen_calc(10, 4,'hamming',0, 0,1,2)  arith_type="Signed  (2's comp)"  n_bits=8  bin_pt=7  latency=3  init_zero=on  explicit_period=off  period=1  rst=off  init_reg=0  en=off  dbl_ovrd=off  show_param=on  distributed_mem=on  use_rpm=on  gen_core=off
      settings: xl_area=[0, 0, 0, 0, 0, 0, 0]
  ROM3 : xbsIndex_r3/ROM  depth=1024  initVector=pfb_coeff_gen_calc(10, 4,'hamming',0, 0,1,3)  arith_type="Signed  (2's comp)"  n_bits=8  bin_pt=7  latency=3  init_zero=on  explicit_period=off  period=1  rst=off  init_reg=0  en=off  dbl_ovrd=off  show_param=off  distributed_mem=on  use_rpm=on  gen_core=off
      settings: xl_area=[0, 0, 0, 0, 0, 0, 0]
  ROM4 : xbsIndex_r3/ROM  depth=1024  initVector=pfb_coeff_gen_calc(10, 4,'hamming',0, 0,1,4)  arith_type="Signed  (2's comp)"  n_bits=8  bin_pt=7  latency=3  init_zero=on  explicit_period=off  period=1  rst=off  init_reg=0  en=off  dbl_ovrd=off  show_param=off  distributed_mem=on  use_rpm=on  gen_core=off
      settings: xl_area=[0, 0, 0, 0, 0, 0, 0]
  Register : xbsIndex_r3/Register  init=0  reg_only_valid=off  explicit_period=off  period=1  rst=off  en=off  out_en=off  dbl_ovrd=off  show_param=off
      settings: xl_area=[0, 0, 0, 0, 0, 0, 0]
  Reinterpret{1..4} (4 alike) : xbsIndex_r3/Reinterpret  force_arith_type=on  arith_type=Unsigned  force_bin_pt=on  bin_pt=0  force_valid=on
  dout : Outport
  sync_out : Outport  Port=2
  coeff : Outport  Port=3
  wires:
  din/1 -> Delay1/1
  Delay1/1 -> dout/1
  sync/1 -> Counter/1, Delay/1
  Delay/1 -> sync_out/1
  Concat/1 -> Register/1
  Register/1 -> coeff/1
  Counter/1 -> ROM1/1, ROM2/1, ROM3/1, ROM4/1
  ROM1/1 -> Reinterpret1/1
  Reinterpret1/1 -> Concat/1
  ROM2/1 -> Reinterpret2/1
  Reinterpret2/1 -> Concat/2
  ROM3/1 -> Reinterpret3/1
  Reinterpret3/1 -> Concat/3
  ROM4/1 -> Reinterpret4/1
  Reinterpret4/1 -> Concat/4

== system dig_int_kurt/pfb_fir/pol2_in1_first_tap/ri_to_c ==
  re : Inport  Port=1  LatchInput=off
  im : Inport  Port=2  LatchInput=off
  Concat : xbsIndex_r3/Concat  num_inputs=2  explicit_period=off  period=1  dbl_ovrd=off
  Reinterpret : xbsIndex_r3/Reinterpret  force_arith_type=on  arith_type=Unsigned  force_bin_pt=on  bin_pt=0  force_valid=on
  Reinterpret1 : xbsIndex_r3/Reinterpret  force_arith_type=on  arith_type=Unsigned  force_bin_pt=on  bin_pt=0  force_valid=on
  c : Outport
  wires:
  Reinterpret/1 -> Concat/1
  Reinterpret1/1 -> Concat/2
  re/1 -> Reinterpret/1
  Concat/1 -> c/1
  im/1 -> Reinterpret1/1

== system dig_int_kurt/pfb_fir/pol2_in1_last_tap/pfb_add_tree ==
  din : Inport  Port=1  LatchInput=off
  sync : Inport  Port=2  LatchInput=off
  Reint0_1 : xbsIndex_r3/Reinterpret  force_arith_type=on  arith_type="Signed  (2's comp)"  force_bin_pt=on  bin_pt=14  force_valid=on
  Reint0_2 : xbsIndex_r3/Reinterpret  force_arith_type=on  arith_type="Signed  (2's comp)"  force_bin_pt=on  bin_pt=14  force_valid=on
  Reint1_1 : xbsIndex_r3/Reinterpret  force_arith_type=on  arith_type="Signed  (2's comp)"  force_bin_pt=on  bin_pt=14  force_valid=on
  Reint1_2 : xbsIndex_r3/Reinterpret  force_arith_type=on  arith_type="Signed  (2's comp)"  force_bin_pt=on  bin_pt=14  force_valid=on
  Reint2_1 : xbsIndex_r3/Reinterpret  force_arith_type=on  arith_type="Signed  (2's comp)"  force_bin_pt=on  bin_pt=14  force_valid=on
  Reint2_2 : xbsIndex_r3/Reinterpret  force_arith_type=on  arith_type="Signed  (2's comp)"  force_bin_pt=on  bin_pt=14  force_valid=on
  Reint3_1 : xbsIndex_r3/Reinterpret  force_arith_type=on  arith_type="Signed  (2's comp)"  force_bin_pt=on  bin_pt=14  force_valid=on
  Reint3_2 : xbsIndex_r3/Reinterpret  force_arith_type=on  arith_type="Signed  (2's comp)"  force_bin_pt=on  bin_pt=14  force_valid=on
  Slice0_1 : xbsIndex_r3/Slice  mode=Upper Bit Location + Width  nbits=16  bit1=0  base1=MSB of Input  bit0=0  base0=MSB of Input  boolean_output=off  explicit_period=off  period=1  dbl_ovrd=off
  Slice0_2 : xbsIndex_r3/Slice  mode=Upper Bit Location + Width  nbits=16  bit1=-16  base1=MSB of Input  bit0=0  base0=MSB of Input  boolean_output=off  explicit_period=off  period=1  dbl_ovrd=off
  Slice1_1 : xbsIndex_r3/Slice  mode=Upper Bit Location + Width  nbits=16  bit1=-32  base1=MSB of Input  bit0=0  base0=MSB of Input  boolean_output=off  explicit_period=off  period=1  dbl_ovrd=off
  Slice1_2 : xbsIndex_r3/Slice  mode=Upper Bit Location + Width  nbits=16  bit1=-48  base1=MSB of Input  bit0=0  base0=MSB of Input  boolean_output=off  explicit_period=off  period=1  dbl_ovrd=off
  Slice2_1 : xbsIndex_r3/Slice  mode=Upper Bit Location + Width  nbits=16  bit1=-64  base1=MSB of Input  bit0=0  base0=MSB of Input  boolean_output=off  explicit_period=off  period=1  dbl_ovrd=off
  Slice2_2 : xbsIndex_r3/Slice  mode=Upper Bit Location + Width  nbits=16  bit1=-80  base1=MSB of Input  bit0=0  base0=MSB of Input  boolean_output=off  explicit_period=off  period=1  dbl_ovrd=off
  Slice3_1 : xbsIndex_r3/Slice  mode=Upper Bit Location + Width  nbits=16  bit1=-96  base1=MSB of Input  bit0=0  base0=MSB of Input  boolean_output=off  explicit_period=off  period=1  dbl_ovrd=off
  Slice3_2 : xbsIndex_r3/Slice  mode=Upper Bit Location + Width  nbits=16  bit1=-112  base1=MSB of Input  bit0=0  base0=MSB of Input  boolean_output=off  explicit_period=off  period=1  dbl_ovrd=off
  adder_tree1 : Subsystem  AncestorBlock=casper_library/Misc/adder_tree  mask(adder_tree){n_inputs=4, latency=2}
      mask prompts: n_inputs "Number of Inputs"; latency "Add Latency"
      mask help: Sums all inputs using a tree of adds and delays.
      mask init:
      | adder_tree_init(gcb, ...
      |     'n_inputs', n_inputs, ...
      |     'latency', latency);
      settings: AttributesFormatString=latency 4
      mask Help: eval('xlWeb([getenv(''MLIB_ROOT''), ''\doc\html\sp_adder_tree\sp_adder_tree.html''])')
  adder_tree2 : Subsystem  AncestorBlock=casper_library/Misc/adder_tree  mask(adder_tree){n_inputs=4, latency=2}
      mask prompts: n_inputs "Number of Inputs"; latency "Add Latency"
      mask help: Sums all inputs using a tree of adds and delays.
      mask init:
      | adder_tree_init(gcb, ...
      |     'n_inputs', n_inputs, ...
      |     'latency', latency);
      settings: AttributesFormatString=latency 4
      mask Help: eval('xlWeb([getenv(''MLIB_ROOT''), ''\doc\html\sp_adder_tree\sp_adder_tree.html''])')
  convert1 : xbsIndex_r3/Convert  arith_type="Signed  (2's comp)"  n_bits=18  bin_pt=17  quantization=Truncate  overflow=Saturate  latency=2  explicit_period=off  period=1  dbl_ovrd=off  show_param=off  inserted_by_tool=off  pipeline=off
      settings: xl_area=[0, 0, 0, 0, 0, 0, 0]
  convert2 : xbsIndex_r3/Convert  arith_type="Signed  (2's comp)"  n_bits=18  bin_pt=17  quantization=Truncate  overflow=Saturate  latency=2  explicit_period=off  period=1  dbl_ovrd=off  show_param=off  inserted_by_tool=off  pipeline=off
      settings: xl_area=[0, 0, 0, 0, 0, 0, 0]
  delay1 : xbsIndex_r3/Delay  latency=2  reg_retiming=off  explicit_period=off  period=1  en=off  accept_only_valid=off  init_zero=on  dbl_ovrd=off  show_param=off
      settings: xl_area=[0, 0, 0, 0, 0, 0, 0]
  ri_to_c : casper_library/Misc/ri_to_c
  scale1 : xbsIndex_r3/Scale  scale_factor=-3  explicit_period=off  period=1  dbl_ovrd=off
  scale2 : xbsIndex_r3/Scale  scale_factor=-3  explicit_period=off  period=1  dbl_ovrd=off
  dout : Outport
  sync_out : Outport  Port=2
  wires:
  adder_tree1/2(dout) -> scale1/1
  scale1/1 -> convert1/1
  adder_tree2/2(dout) -> scale2/1
  scale2/1 -> convert2/1
  convert1/1 -> ri_to_c/1
  convert2/1 -> ri_to_c/2
  ri_to_c/1 -> dout/1
  sync/1 -> adder_tree1/1(sync), adder_tree2/1(sync)
  adder_tree1/1(sync_out) -> delay1/1
  delay1/1 -> sync_out/1
  din/1 -> Slice0_1/1, Slice0_2/1, Slice1_1/1, Slice1_2/1, Slice2_1/1, Slice2_2/1, Slice3_1/1, Slice3_2/1
  Slice0_1/1 -> Reint0_1/1
  Reint0_1/1 -> adder_tree1/2(din1)
  Slice0_2/1 -> Reint0_2/1
  Reint0_2/1 -> adder_tree2/2(din1)
  Slice1_1/1 -> Reint1_1/1
  Reint1_1/1 -> adder_tree1/3(din2)
  Slice1_2/1 -> Reint1_2/1
  Reint1_2/1 -> adder_tree2/3(din2)
  Slice2_1/1 -> Reint2_1/1
  Reint2_1/1 -> adder_tree1/4(din3)
  Slice2_2/1 -> Reint2_2/1
  Reint2_2/1 -> adder_tree2/4(din3)
  Slice3_1/1 -> Reint3_1/1
  Reint3_1/1 -> adder_tree1/5(din4)
  Slice3_2/1 -> Reint3_2/1
  Reint3_2/1 -> adder_tree2/5(din4)

== system dig_int_kurt/pfb_fir/pol2_in1_last_tap/ri_to_c ==
  re : Inport  Port=1  LatchInput=off
  im : Inport  Port=2  LatchInput=off
  Concat : xbsIndex_r3/Concat  num_inputs=2  explicit_period=off  period=1  dbl_ovrd=off
  Reinterpret : xbsIndex_r3/Reinterpret  force_arith_type=on  arith_type=Unsigned  force_bin_pt=on  bin_pt=0  force_valid=on
  Reinterpret1 : xbsIndex_r3/Reinterpret  force_arith_type=on  arith_type=Unsigned  force_bin_pt=on  bin_pt=0  force_valid=on
  c : Outport
  wires:
  im/1 -> Reinterpret1/1
  Concat/1 -> c/1
  re/1 -> Reinterpret/1
  Reinterpret1/1 -> Concat/2
  Reinterpret/1 -> Concat/1
